simulink model "Ideal_R2017b"  (R2017a)
settings: Solver=ode4  StartTime=0  StopTime=1200  FixedStep=0.1  MaxStep=0.05  RelTol=1e-5
values from neighbouring files (symbols this model uses):
  Av = 1.725*1.490    (= 2.57025)    [Ideal_initiate.m]
  Cd = 0.26    [Ideal_initiate.m]
  Cr = 0.008    [Ideal_initiate.m]
  Density = (85*19.6e6 + 15*32e6)/100    (= 21460000)    [Ideal_initiate.m]
  grav = 9.81    [Ideal_initiate.m]
  Mv = (1325 + 250)    (= 1575)    [Ideal_initiate.m]
  rho_air = 1.225    [Ideal_initiate.m]
  rw = 0.30    (= 0.3)    [Ideal_initiate.m]
  T_max = inf    [Ideal_initiate.m]
  T_min = 0    [Ideal_initiate.m]
settings Model: ExtModeTrigMode=oneshot  ExtModeArmWhenConnect=off  Creator=leksell  LastModifiedBy=Callum
settings DataIOCC: SaveFormat=Array  SignalLoggingSaveFormat=ModelDataLogs  SignalLoggingName=sigsOut
settings OptimizationCC: BlockReduction=off  BooleanDataType=off  ExpressionDepthLimit=2147483647  InitFltsAndDblsToZero=on  LifeSpan=inf
settings DebuggingCC: ConsistencyChecking=warning  SaveWithParameterizedLinksMsg=none  UnderspecifiedInitializationDetection=Classic  MergeDetectMultiDrivingBlocksExec=none  SignalResolutionControl=TryResolveAllWithWarning  MultiTaskDSMMsg=warning  MultiTaskCondExecSysMsg=none  UnnecessaryDatatypeConvMsg=warning  FcnCallInpInsideContextMsg=warning  UnconnectedInputMsg=none  UnconnectedOutputMsg=none  UnconnectedLineMsg=none  AllowSymbolicDim=off  StateNameClashWarn=warning  SFUnexpectedBacktrackingDiag=warning  SFNoUnconditionalDefaultTransitionDiag=warning  SFExecutionAtInitializationDiag=none
settings HardwareCC: ProdBitPerPointer=32  ProdBitPerSizeT=32  ProdBitPerPtrDiffT=32  ProdLargestAtomicFloat=None  ProdIntDivRoundTo=Undefined  ProdEndianess=Unspecified  ProdWordSize=32  ProdHWDeviceType=32-bit Generic  TargetUnknown=on
settings ModelReferenceCC: PropagateSignalLabelsOutOfModel=off
settings GRTTargetCC: TargetFcnLib=ansi_tfl_tmw.mat  TargetLangStandard=C89/C90 (ANSI)  GeneratePreprocessorConditionals=Disable all  CombineOutputUpdateFcns=off  GRTInterface=on
settings ConfigComp: CovMetricSettings=dw  CovHtmlReporting=on  CovSaveCumulativeToWorkspaceVar=on  CovSaveSingleToWorkspaceVar=on  CovExternalEMLEnable=off

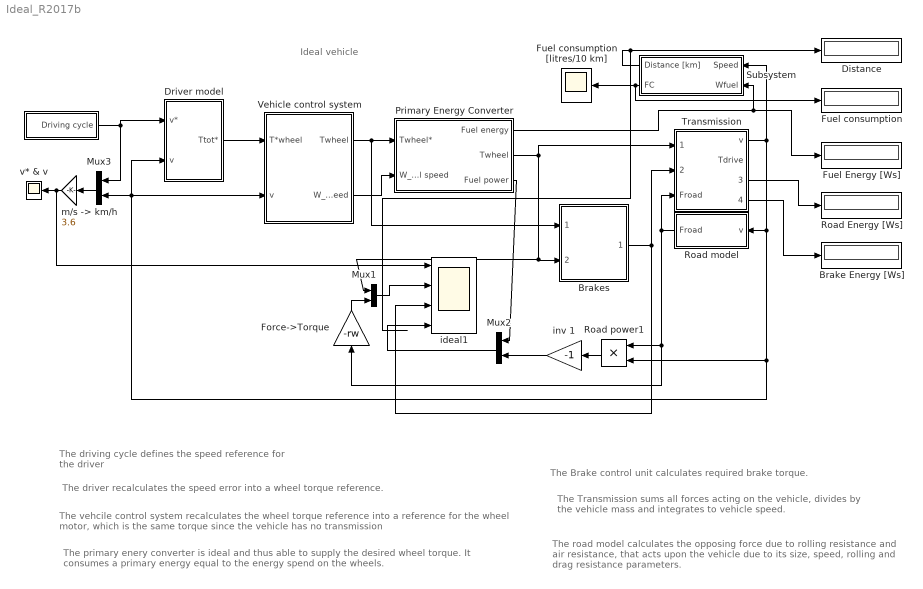
== system Ideal_R2017b ==
  note: Ideal vehicle
  note: The driving cycle defines the speed reference
      | for the driver
  note: The vehcile control system recalculates the wheel torque reference into a reference for the wheel
      | motor, which is the same torque since the vehicle has no transmission
  note: The primary enery converter is ideal and thus able to supply the desired wheel torque.
      | It consumes a primary energy equal to the energy spend on the wheels.
  note: The Brake control unit calculates required brake torque.
  note: The Transmission sums all forces acting on the vehicle, divides
      | by the vehicle mass and integrates to vehicle speed.
  note: The driver recalculates the speed error into a wheel torque reference.
  note: The road model calculates the opposing force due to rolling resistance
      | and air resistance, that acts upon the vehicle due to its size, speed,
      | rolling and drag resistance parameters.
  " " : Subsystem  mask{Cycle=IdealMotion}
      mask prompts: Cycle "Driving cycle"
      mask TypeOptions Cycle: nedc | us06 | IdealMotion
  Brake Energy [Ws] : Display
  Brakes : Subsystem
  Distance : Display
  "Driver model " : Subsystem  mask{Mv=Mv, rw=rw, T_max=T_max}
      mask prompts: Mv "Vehicle Mass"; rw "Wheel Radius"; T_max "Max Wheel Torque"
      mask init:
      | Ti = 3 + 7*(Mv-1000)/9000;
      | Kv=4*Mv/Ti;
  Force->Torque : Gain  Gain=-rw  SaturateOnIntegerOverflow=on  OutDataTypeStr=Inherit: Same as input  ParamDataTypeStr=Inherit: Same as input
  Fuel Energy [Ws] : Display
  Fuel consumption : Display
  Fuel consumption [litres/10 km] : Scope
  Mux1 : Mux  Inputs=2
  Mux2 : Mux  Inputs=2
  Mux3 : Mux  Inputs=2
  Primary Energy Converter : Subsystem
  Road Energy [Ws] : Display
  Road model : Subsystem
  Road power1 : Product  Inputs=**  SaturateOnIntegerOverflow=on  InputSameDT=on  OutDataTypeStr=Inherit: Same as first input
  Subsystem : Subsystem
  Transmission : Subsystem
  Vehicle control system : Subsystem
  ideal1 : Scope  NumInputPorts=4
  inv 1 : Gain  Gain=-1  SaturateOnIntegerOverflow=on  OutDataTypeStr=Inherit: Same as input  ParamDataTypeStr=Inherit: Same as input
  "m/s -> km/h" : Gain  Gain=3.6  SaturateOnIntegerOverflow=on  OutDataTypeStr=Inherit: Same as input  ParamDataTypeStr=Inherit: Same as input
  v* & v : Scope
  wires:
  Primary Energy Converter/2(Twheel) -> Transmission/1(Twheel), Mux1/1, Brakes/2(Twheel)
  " "/1(Driving cycle) -> Mux3/1, "Driver model "/1(v*)
  "Driver model "/1(Ttot*) -> Vehicle control system/1(T*wheel)
  Mux3/1 -> "m/s -> km/h"/1
  Vehicle control system/1(Twheel) -> Primary Energy Converter/1(Twheel*), Brakes/1(T*wheel)
  Transmission/1(v) -> Road power1/2, Mux3/2, "Driver model "/2(v), Vehicle control system/2(v), Road model/1("v "), Subsystem/1(Speed)
  Road model/1(Froad) -> Transmission/3(Froad), Road power1/1, Force->Torque/1
  Brakes/1(T_brake) -> Transmission/2(Tbrake), ideal1/3
  Primary Energy Converter/1(Fuel energy) -> Subsystem/2(Wfuel), Fuel Energy [Ws]/1
  "m/s -> km/h"/1 -> ideal1/1, v* & v/1
  Transmission/3(Wfriction) -> Road Energy [Ws]/1
  Transmission/4(Wbrake) -> Brake Energy [Ws]/1
  Vehicle control system/2(W_wheel speed) -> Primary Energy Converter/2(W_wheel speed)
  Mux1/1 -> ideal1/2
  Force->Torque/1 -> Mux1/2
  Subsystem/1(Distance [km]) -> Distance/1
  Mux2/1 -> ideal1/4
  Primary Energy Converter/3("Fuel power ") -> Mux2/1
  Road power1/1 -> inv 1/1
  inv 1/1 -> Mux2/2
  Subsystem/2(FC) -> Fuel consumption/1, Fuel consumption [litres/10 km]/1

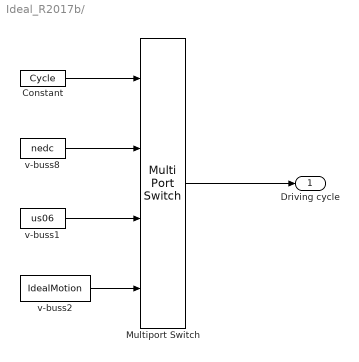
== system Ideal_R2017b/  ==
  Constant : Constant  Value=Cycle
  Multiport Switch : MultiPortSwitch  SaturateOnIntegerOverflow=on  InputSameDT=on
  v-buss1 : FromWorkspace  VariableName=us06  SampleTime=.1
  v-buss2 : FromWorkspace  VariableName=IdealMotion  SampleTime=.1
  v-buss8 : FromWorkspace  VariableName=nedc  SampleTime=.1
  Driving cycle : Outport
  wires:
  v-buss8/1 -> Multiport Switch/2
  Constant/1 -> Multiport Switch/1
  v-buss1/1 -> Multiport Switch/3
  v-buss2/1 -> Multiport Switch/4
  Multiport Switch/1 -> Driving cycle/1

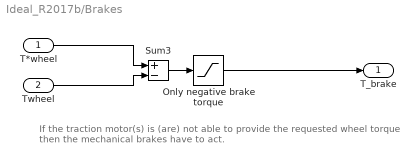
== system Ideal_R2017b/Brakes ==
  note: If the traction motor(s) is (are) not able to provide the requested wheel torque
      | then the mechanical brakes have to act.
  T*wheel : Inport
  Twheel : Inport  Port=2
  Only negative brake torque : Saturate  UpperLimit=0  LowerLimit=-inf
  Sum3 : Sum  Inputs=+-  SaturateOnIntegerOverflow=on  InputSameDT=on  OutDataTypeStr=Inherit: Same as first input
  T_brake : Outport  InitialOutput=0
  wires:
  Sum3/1 -> Only negative brake torque/1
  T*wheel/1 -> Sum3/1
  Twheel/1 -> Sum3/2
  Only negative brake torque/1 -> T_brake/1

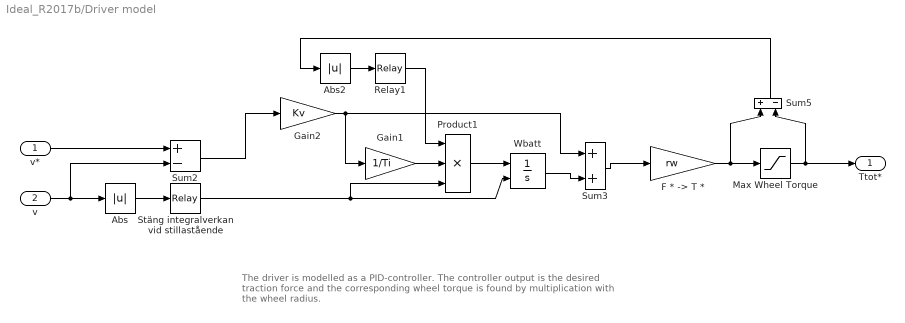
== system Ideal_R2017b/Driver model  ==
  note: The driver is modelled as a PID-controller.
      | The controller output is the desired traction force and the
      | corresponding wheel torque is found by multiplication with the wheel radius.
  v* : Inport
  v : Inport  Port=2
  Abs : Abs  SaturateOnIntegerOverflow=on
  Abs2 : Abs  SaturateOnIntegerOverflow=on
  "F * -> T *" : Gain  Gain=rw  SaturateOnIntegerOverflow=on  OutDataTypeStr=Inherit: Same as input  ParamDataTypeStr=Inherit: Same as input
  Gain1 : Gain  Gain=1/Ti  SaturateOnIntegerOverflow=on  OutDataTypeStr=Inherit: Same as input  ParamDataTypeStr=Inherit: Same as input
  Gain2 : Gain  Gain=Kv  SaturateOnIntegerOverflow=on  OutDataTypeStr=Inherit: Same as input  ParamDataTypeStr=Inherit: Same as input
  Max Wheel Torque : Saturate  UpperLimit=T_max  LowerLimit=-T_max
  Product1 : Product  Inputs=3  SaturateOnIntegerOverflow=on  InputSameDT=on  OutDataTypeStr=Inherit: Same as first input
  Relay1 : Relay  OnOutputValue=0  OffOutputValue=1
  Stäng integralverkan vid stillastående : Relay  OnSwitchValue=0.3  OffSwitchValue=0.3-eps
  Sum2 : Sum  Inputs=+-  SaturateOnIntegerOverflow=on  InputSameDT=on  OutDataTypeStr=Inherit: Same as first input
  Sum3 : Sum  SaturateOnIntegerOverflow=on  InputSameDT=on  OutDataTypeStr=Inherit: Same as first input
  Sum5 : Sum  Inputs=+-  SaturateOnIntegerOverflow=on  InputSameDT=on  OutDataTypeStr=Inherit: Same as first input
  Wbatt : Integrator  ExternalReset=falling  LimitOutput=on  UpperSaturationLimit=1000  LowerSaturationLimit=-10000
  Ttot* : Outport  InitialOutput=0
  wires:
  v/1 -> Sum2/2, Abs/1
  v*/1 -> Sum2/1
  Sum2/1 -> Gain2/1
  Stäng integralverkan vid stillastående/1 -> Wbatt/2, Product1/3
  Gain2/1 -> Sum3/1, Gain1/1
  "F * -> T *"/1 -> Max Wheel Torque/1, Sum5/1
  Wbatt/1 -> Sum3/2
  Sum3/1 -> "F * -> T *"/1
  Product1/1 -> Wbatt/1
  Abs/1 -> Stäng integralverkan vid stillastående/1
  Gain1/1 -> Product1/2
  Abs2/1 -> Relay1/1
  Relay1/1 -> Product1/1
  Max Wheel Torque/1 -> Ttot*/1, Sum5/2
  Sum5/1 -> Abs2/1

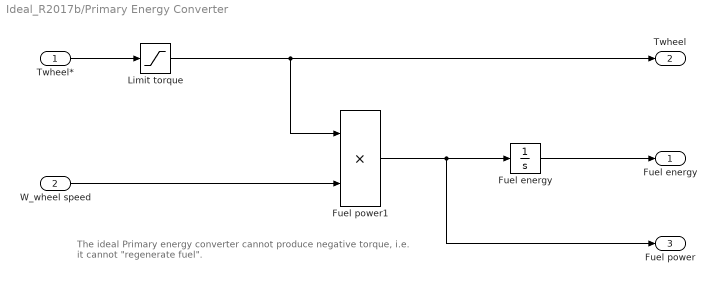
== system Ideal_R2017b/Primary Energy Converter ==
  note: The ideal Primary energy converter cannot produce negative torque,
      | i.e. it cannot "regenerate fuel".
  Twheel* : Inport
  W_wheel speed : Inport  Port=2
  "Fuel energy " : Integrator
  Fuel power1 : Product  Inputs=**  SaturateOnIntegerOverflow=on  InputSameDT=on  OutDataTypeStr=Inherit: Same as first input
  Limit torque : Saturate  UpperLimit=T_max  LowerLimit=T_min
  Fuel energy : Outport  InitialOutput=0
  Twheel : Outport  Port=2  InitialOutput=0
  "Fuel power " : Outport  Port=3  InitialOutput=0
  wires:
  "Fuel energy "/1 -> Fuel energy/1
  Twheel*/1 -> Limit torque/1
  Limit torque/1 -> Twheel/1, Fuel power1/1
  W_wheel speed/1 -> Fuel power1/2
  Fuel power1/1 -> "Fuel power "/1, "Fuel energy "/1

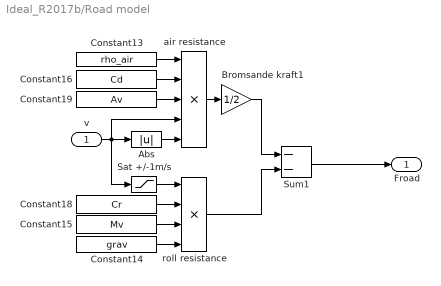
== system Ideal_R2017b/Road model ==
  "v " : Inport
  Abs : Abs  SaturateOnIntegerOverflow=on
  Bromsande kraft1 : Gain  Gain=1/2  SaturateOnIntegerOverflow=on  OutDataTypeStr=Inherit: Same as input  ParamDataTypeStr=Inherit: Same as input
  Constant13 : Constant  Value=rho_air
  Constant14 : Constant  Value=grav
  Constant15 : Constant  Value=Mv
  Constant16 : Constant  Value=Cd
  Constant18 : Constant  Value=Cr
  Constant19 : Constant  Value=Av
  Sat +/-1m/s : Saturate  UpperLimit=1  LowerLimit=-1
  Sum1 : Sum  Inputs=--  SaturateOnIntegerOverflow=on  InputSameDT=on  OutDataTypeStr=Inherit: Same as first input
  air resistance : Product  Inputs=5  SaturateOnIntegerOverflow=on  InputSameDT=on  OutDataTypeStr=Inherit: Same as first input
  roll resistance : Product  Inputs=4  SaturateOnIntegerOverflow=on  InputSameDT=on  OutDataTypeStr=Inherit: Same as first input
  Froad : Outport  InitialOutput=0
  wires:
  air resistance/1 -> Bromsande kraft1/1
  Sum1/1 -> Froad/1
  Bromsande kraft1/1 -> Sum1/1
  roll resistance/1 -> Sum1/2
  Constant13/1 -> air resistance/1
  Constant16/1 -> air resistance/2
  Constant19/1 -> air resistance/3
  "v "/1 -> air resistance/4, Sat +/-1m/s/1, Abs/1
  Constant18/1 -> roll resistance/2
  Constant15/1 -> roll resistance/3
  Constant14/1 -> roll resistance/4
  Sat +/-1m/s/1 -> roll resistance/1
  Abs/1 -> air resistance/5

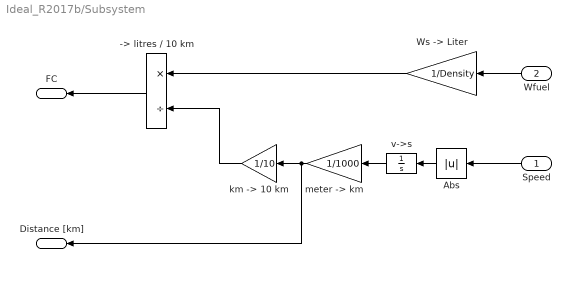
== system Ideal_R2017b/Subsystem ==
  Speed : Inport
  Wfuel : Inport  Port=2
  -> litres / 10 km : Product  Inputs=*/  SaturateOnIntegerOverflow=on  InputSameDT=on  OutDataTypeStr=Inherit: Same as first input
  Abs : Abs  SaturateOnIntegerOverflow=on
  "Ws -> Liter" : Gain  Gain=1/Density  SaturateOnIntegerOverflow=on  OutDataTypeStr=Inherit: Same as input  ParamDataTypeStr=Inherit: Same as input
  "km -> 10 km" : Gain  Gain=1/10  SaturateOnIntegerOverflow=on  OutDataTypeStr=Inherit: Same as input  ParamDataTypeStr=Inherit: Same as input
  "meter -> km" : Gain  Gain=1/1000  SaturateOnIntegerOverflow=on  OutDataTypeStr=Inherit: Same as input  ParamDataTypeStr=Inherit: Same as input
  v->s : Integrator  InitialCondition=1  LimitOutput=on
  Distance [km] : Outport
  FC : Outport  Port=2
  wires:
  "Ws -> Liter"/1 -> -> litres / 10 km/1
  v->s/1 -> "meter -> km"/1
  -> litres / 10 km/1 -> FC/1
  Wfuel/1 -> "Ws -> Liter"/1
  Speed/1 -> Abs/1
  "meter -> km"/1 -> Distance [km]/1, "km -> 10 km"/1
  Abs/1 -> v->s/1
  "km -> 10 km"/1 -> -> litres / 10 km/2

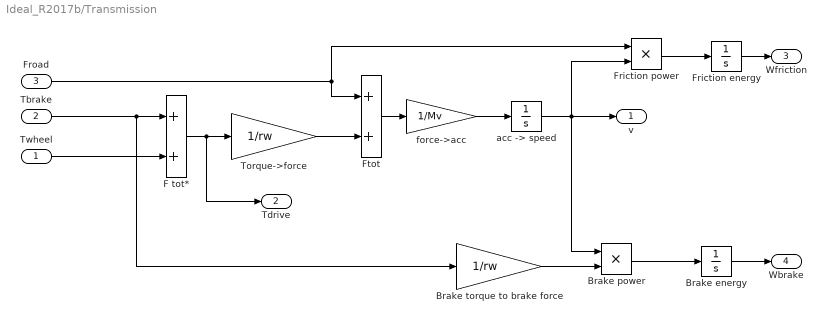
== system Ideal_R2017b/Transmission ==
  Twheel : Inport
  Tbrake : Inport  Port=2
  Froad : Inport  Port=3
  Brake energy : Integrator
  "Brake power " : Product  SaturateOnIntegerOverflow=on  InputSameDT=on  OutDataTypeStr=Inherit: Same as first input
  Brake torque to brake force : Gain  Gain=1/rw  SaturateOnIntegerOverflow=on  OutDataTypeStr=Inherit: Same as input  ParamDataTypeStr=Inherit: Same as input
  F tot* : Sum  SaturateOnIntegerOverflow=on  InputSameDT=on  OutDataTypeStr=Inherit: Same as first input
  Friction energy : Integrator
  Friction power : Product  SaturateOnIntegerOverflow=on  InputSameDT=on  OutDataTypeStr=Inherit: Same as first input
  Ftot : Sum  SaturateOnIntegerOverflow=on  InputSameDT=on  OutDataTypeStr=Inherit: Same as first input
  Torque->force : Gain  Gain=1/rw  SaturateOnIntegerOverflow=on  OutDataTypeStr=Inherit: Same as input  ParamDataTypeStr=Inherit: Same as input
  "acc -> speed" : Integrator
  force->acc : Gain  Gain=1/Mv  SaturateOnIntegerOverflow=on  OutDataTypeStr=Inherit: Same as input  ParamDataTypeStr=Inherit: Same as input
  v : Outport  InitialOutput=0
  Tdrive : Outport  Port=2  InitialOutput=0
  Wfriction : Outport  Port=3  InitialOutput=0
  Wbrake : Outport  Port=4  InitialOutput=0
  wires:
  force->acc/1 -> "acc -> speed"/1
  Twheel/1 -> F tot*/2
  "acc -> speed"/1 -> v/1, "Brake power "/1, Friction power/2
  F tot*/1 -> Torque->force/1, Tdrive/1
  Tbrake/1 -> F tot*/1, Brake torque to brake force/1
  Torque->force/1 -> Ftot/2
  Ftot/1 -> force->acc/1
  Froad/1 -> Ftot/1, Friction power/1
  Brake torque to brake force/1 -> "Brake power "/2
  "Brake power "/1 -> Brake energy/1
  Friction power/1 -> Friction energy/1
  Friction energy/1 -> Wfriction/1
  Brake energy/1 -> Wbrake/1

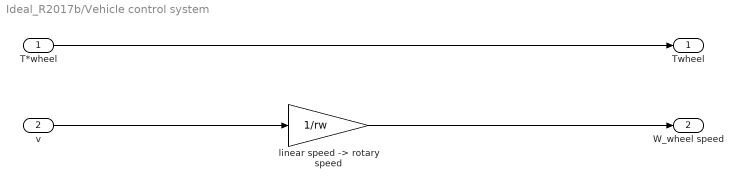
== system Ideal_R2017b/Vehicle control system ==
  T*wheel : Inport
  v : Inport  Port=2
  "linear speed -> rotary speed" : Gain  Gain=1/rw  SaturateOnIntegerOverflow=on  OutDataTypeStr=Inherit: Same as input  ParamDataTypeStr=Inherit: Same as input
  Twheel : Outport
  W_wheel speed : Outport  Port=2
  wires:
  T*wheel/1 -> Twheel/1
  v/1 -> "linear speed -> rotary speed"/1
  "linear speed -> rotary speed"/1 -> W_wheel speed/1
